simulink model "sim_MSDSystem_eg2"  (R2021b)
settings: Solver=VariableStepAuto  StartTime=0.0  StopTime=10.0  RelTol=1e-3
values from neighbouring files (symbols this model uses):
  c = 3    [MSDSystem_eg2.m]
  F = 10    [MSDSystem_eg2.m]
  k = 20    [MSDSystem_eg2.m]    (also in Pendulum_hangingFromHarmonicOscillator.m)
  m = 10    [MSDSystem_eg1.m]    (also in MSDSystem_eg2.m = 4; Pendulum_hangingFromHarmonicOscillator.m = 200; Pendulum_withFreeSupport.m = 200)
settings Model: Creator=Samir  LastModifiedBy=Samir

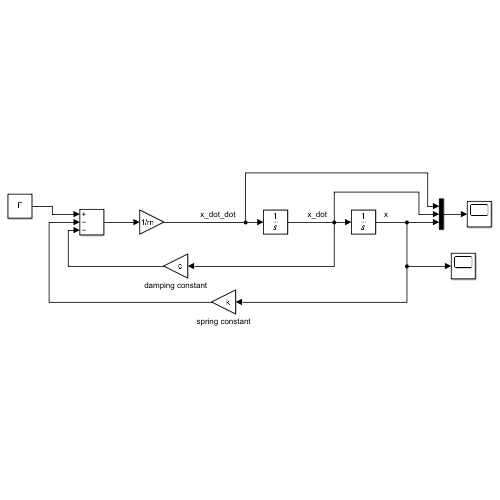
[thumbnail: Simulink's stored preview of the top-level diagram]
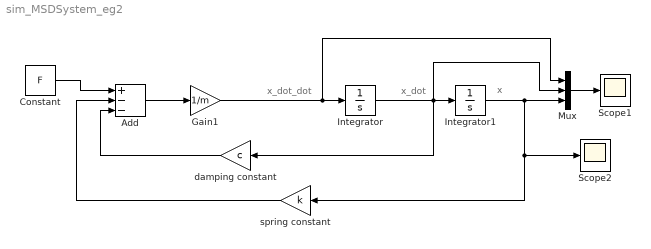
== system sim_MSDSystem_eg2 ==
  note: x
  note: x_dot
  note: x_dot_dot
  Add : Sum  Inputs=+--
  Constant : Constant  Value=F
  Gain1 : Gain  Gain=1/m
  Integrator : Integrator
  Integrator1 : Integrator
  Mux : Mux  Inputs=3
  Scope1 : Scope
  Scope2 : Scope
  damping constant : Gain  Gain=c
  spring constant : Gain  Gain=k
  wires:
  Integrator/1 -> damping constant/1, Mux/2, Integrator1/1
  Add/1 -> Gain1/1
  Gain1/1 -> Mux/1, Integrator/1
  Constant/1 -> Add/1
  damping constant/1 -> Add/3
  spring constant/1 -> Add/2
  Integrator1/1 -> spring constant/1, Scope2/1, Mux/3
  Mux/1 -> Scope1/1
